simulink model "Vector_Calculator"  (R2021a)
settings: Solver=VariableStepAuto  StartTime=0.0  StopTime=10.0  RelTol=1e-3
libraries: dspmtrx3 x1
settings Model: Creator=Nour  LastModifiedBy=Nour

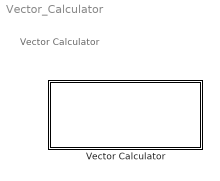
== system Vector_Calculator ==
  note: Vector Calculator
  Vector Calculator : Subsystem

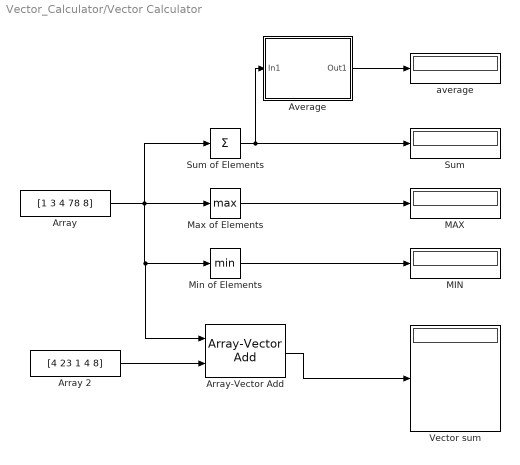
== system Vector_Calculator/Vector Calculator ==
  "Array " : Constant  Value=[1 3 4 78 8]  OutDataTypeStr=double
  Array 2 : Constant  Value=[4 23 1 4 8]  OutDataTypeStr=double
  Array-Vector Add : dspmtrx3/Array-Vector Add  Dimension=1  V_Source=Input port  V_VectFromMask=[0.5 0.25]  prodOutputSignedness=Auto  roundingMode=Floor  overflowMode=off  firstCoeffSignedness=Auto  firstCoeffDataTypeStr=Inherit: Same word length as input  firstCoeffMin=[]  firstCoeffMax=[]  firstCoeffLastDataTypeStr=Inherit: Same word length as input  accumSignedness=Auto  outputSignedness=Auto  outputDataTypeStr=Inherit: Same as accumulator  outputMin=[]  outputMax=[]  outputLastDataTypeStr=Inherit: Same as accumulator
      settings: SourceProductBaseCode=DS
  Average : Subsystem
  MAX : Display
  MIN : Display
  Max of Elements : MinMax  Function=max
  Min of Elements : MinMax
  Sum : Display
  Sum of Elements : Sum  Inputs=+
  Vector sum : Display
  average : Display
  wires:
  Array-Vector Add/1 -> Vector sum/1
  Sum of Elements/1 -> Average/1(In1), Sum/1
  "Array "/1 -> Sum of Elements/1, Array-Vector Add/1, Min of Elements/1, Max of Elements/1
  Max of Elements/1 -> MAX/1
  Min of Elements/1 -> MIN/1
  Array 2/1 -> Array-Vector Add/2
  Average/1(Out1) -> average/1

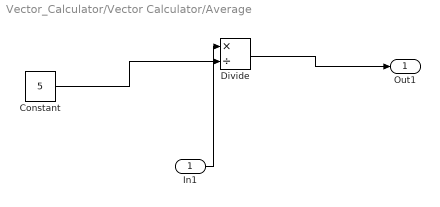
== system Vector_Calculator/Vector Calculator/Average ==
  In1 : Inport
  Constant : Constant  Value=5
  Divide : Product  Inputs=*/
  Out1 : Outport
  wires:
  Constant/1 -> Divide/2
  Divide/1 -> Out1/1
  In1/1 -> Divide/1
